simulink model "HighClearance_model"  (R2019b)
settings: configuration reference "configRef" (kept outside this file)
undefined symbols (not defined in the file): baseClearance, calSTEP1_e, calSTEP2_e, calSTEP3_e, calSTEP4_e, calTolMultiplier, errorMinSpd, heightCalibrating_e, heightDiffTolerance, heightDown_e, heightError_e, heightMovingDown_e, heightMovingUp_e, heightUnknown_e, heightUp_e, IOD_OK, IOD_Open, IOD_ScGnd, maxMedianWheelAngle, maxTransitionMachineSpd, minTransitionMachineSpd, positionSensor_tblData, positionSensorFL_BrkPnts, positionSensorFR_BrkPnts, positionSensorRL_BrkPnts, positionSensorRR_BrkPnts, step_time, trackWidthMax, trackWidthMin, trackWidthTolerance, twoWheelSteer
libraries: HighClearance_library x129, simulink x25
(part 2 of 3)

== system HighClearance_model/Inputs/clyCoilDiagsLatchLogic ==
  cylCoilDiags : Inport  OutDataTypeStr=Bus: CoilStateBus
  coilStateBreakOut : HighClearance_library/coilStateBreakOut  SystemSampleTime=-1  Latency=0  AutoFrameSizeCalculation=off
  coilStateBus : HighClearance_library/coilStateBus  SystemSampleTime=-1  Latency=0  AutoFrameSizeCalculation=off
  diagLatch{,1..7} (8 alike) : HighClearance_library/diagLatch  SystemSampleTime=-1  Latency=0  AutoFrameSizeCalculation=off
  cylCoilDiagsLatched : Outport  OutDataTypeStr=Bus: CoilStateBus
  wires:
  cylCoilDiags/1 -> coilStateBreakOut/1
  coilStateBreakOut/1 -> diagLatch/1
  diagLatch/1 -> coilStateBus/1
  coilStateBreakOut/2 -> diagLatch1/1
  diagLatch1/1 -> coilStateBus/2
  coilStateBreakOut/3 -> diagLatch2/1
  diagLatch2/1 -> coilStateBus/3
  coilStateBreakOut/5 -> diagLatch4/1
  diagLatch4/1 -> coilStateBus/5
  coilStateBreakOut/7 -> diagLatch6/1
  diagLatch6/1 -> coilStateBus/7
  coilStateBreakOut/4 -> diagLatch3/1
  coilStateBreakOut/6 -> diagLatch5/1
  coilStateBreakOut/8 -> diagLatch7/1
  diagLatch3/1 -> coilStateBus/4
  diagLatch5/1 -> coilStateBus/6
  diagLatch7/1 -> coilStateBus/8
  coilStateBus/1 -> cylCoilDiagsLatched/1

== system HighClearance_model/Inputs/legPositions ==
  positionSensors_mA : Inport  OutDataTypeStr=Bus: CylinderBus
  posSensorCalOkay : Inport  Port=2
  heightPosSensors_diag : Inport  Port=3  OutDataTypeStr=Bus: StateBus
  engRunning : Inport  Port=4  OutDataTypeStr=boolean
  Switch : Switch  Criteria=u2 > Threshold
  calibratedPositions : Subsystem
  checkPlausiLogic : Subsystem
  posSensorCalOkay1 : InportShadow  Port=2
  positionFilterLogic : HighClearance_library/positionFilterLogic  SystemSampleTime=-1  Latency=0  AutoFrameSizeCalculation=off
  positionPlausibilityCheck : Subsystem
  postionToClearance : HighClearance_library/postionToClearance  SystemSampleTime=-1  Latency=0  AutoFrameSizeCalculation=off
  uncalibratedPositions : HighClearance_library/uncalibratedPositions  SystemSampleTime=-1  Latency=0  AutoFrameSizeCalculation=off
  legClearance_mm : Outport  OutDataTypeStr=Bus: CylinderBus
  clyPositionsRaw_mm : Outport  Port=2  OutDataTypeStr=Bus: CylinderBus
  clyPositionsFlt_mm : Outport  Port=3  OutDataTypeStr=Bus: CylinderBus
  heightPosDiagsLatched : Outport  Port=4  OutDataTypeStr=Bus: StateBus
  wires:
  calibratedPositions/1(cylPos_mm) -> Switch/1
  posSensorCalOkay/1 -> Switch/2
  uncalibratedPositions/1 -> Switch/3
  Switch/1 -> positionPlausibilityCheck/2(posIn)
  positionSensors_mA/1 -> uncalibratedPositions/1, calibratedPositions/1(cylPos_mA)
  heightPosSensors_diag/1 -> postionToClearance/3
  postionToClearance/1 -> legClearance_mm/1
  positionFilterLogic/2 -> postionToClearance/1
  positionFilterLogic/1 -> clyPositionsFlt_mm/1
  postionToClearance/2 -> heightPosDiagsLatched/1
  positionPlausibilityCheck/1(posOut) -> positionFilterLogic/1, clyPositionsRaw_mm/1
  positionPlausibilityCheck/2(plausiErr) -> postionToClearance/2
  posSensorCalOkay1/1 -> checkPlausiLogic/1(posSensorCalOkay)
  engRunning/1 -> checkPlausiLogic/2(engRunning)
  checkPlausiLogic/1(enablePlausiCheck) -> positionPlausibilityCheck/1(enablePlausiCheck)

== system HighClearance_model/Inputs/trackCylCoilDiagsLatchLogic ==
  trackCylCoilDiags : Inport  OutDataTypeStr=Bus: CoilStateBus
  coilStateBreakOut : HighClearance_library/coilStateBreakOut  SystemSampleTime=-1  Latency=0  AutoFrameSizeCalculation=off
  coilStateBus : HighClearance_library/coilStateBus  SystemSampleTime=-1  Latency=0  AutoFrameSizeCalculation=off
  diagLatch{,1..7} (8 alike) : HighClearance_library/diagLatch  SystemSampleTime=-1  Latency=0  AutoFrameSizeCalculation=off
  trackCylCoilDiagsLatched : Outport  OutDataTypeStr=Bus: CoilStateBus
  wires:
  coilStateBreakOut/1 -> diagLatch/1
  diagLatch/1 -> coilStateBus/1
  coilStateBreakOut/2 -> diagLatch1/1
  diagLatch1/1 -> coilStateBus/2
  coilStateBreakOut/3 -> diagLatch2/1
  diagLatch2/1 -> coilStateBus/3
  coilStateBreakOut/5 -> diagLatch4/1
  diagLatch4/1 -> coilStateBus/5
  coilStateBreakOut/7 -> diagLatch6/1
  diagLatch6/1 -> coilStateBus/7
  coilStateBreakOut/4 -> diagLatch3/1
  coilStateBreakOut/6 -> diagLatch5/1
  coilStateBreakOut/8 -> diagLatch7/1
  diagLatch3/1 -> coilStateBus/4
  diagLatch5/1 -> coilStateBus/6
  diagLatch7/1 -> coilStateBus/8
  trackCylCoilDiags/1 -> coilStateBreakOut/1
  coilStateBus/1 -> trackCylCoilDiagsLatched/1

== system HighClearance_model/Calibration/controlLogic/calStateConverstion ==
  calState : Inport
  calState2TargetState : Stateflow chart  TreatAsAtomicUnit=on
  targetState : Outport
  wires:
  calState/1 -> calState2TargetState/1(calState)
  calState2TargetState/1(targetState) -> targetState/1

== system HighClearance_model/Calibration/controlLogic/enableCoils ==
  coilDutyCycle : Inport
  enables : Inport  Port=2  OutDataTypeStr=Bus: StateBus
  Bus Selector : BusSelector  OutputSignals=FrontLeft,FrontRight,RearLeft,RearRight
  coilBreakOut : HighClearance_library/coilBreakOut  SystemSampleTime=-1  Latency=0  AutoFrameSizeCalculation=off
  coilBus : HighClearance_library/coilBus  SystemSampleTime=-1  Latency=0  AutoFrameSizeCalculation=off
  passThroughLogic{,1..7} (8 alike) : HighClearance_library/passThroughLogic  SystemSampleTime=-1  Latency=0  AutoFrameSizeCalculation=off
  coilDutyCycle_pct : Outport  OutDataTypeStr=Bus: CoilBus
  wires:
  coilDutyCycle/1 -> coilBreakOut/1
  enables/1 -> Bus Selector/1
  coilBus/1 -> coilDutyCycle_pct/1
  coilBreakOut/1 -> passThroughLogic/1
  Bus Selector/1 -> passThroughLogic1/2, passThroughLogic/2  "<FrontLeft>"
  coilBreakOut/2 -> passThroughLogic1/1
  passThroughLogic1/1 -> coilBus/2
  passThroughLogic/1 -> coilBus/1
  passThroughLogic5/1 -> coilBus/6
  passThroughLogic6/1 -> coilBus/7
  passThroughLogic4/1 -> coilBus/5
  passThroughLogic7/1 -> coilBus/8
  passThroughLogic3/1 -> coilBus/4
  passThroughLogic2/1 -> coilBus/3
  coilBreakOut/3 -> passThroughLogic2/1
  Bus Selector/2 -> passThroughLogic3/2, passThroughLogic2/2  "<FrontRight>"
  Bus Selector/3 -> passThroughLogic5/2, passThroughLogic4/2  "<RearLeft>"
  Bus Selector/4 -> passThroughLogic6/2, passThroughLogic7/2  "<RearRight>"
  coilBreakOut/4 -> passThroughLogic3/1
  coilBreakOut/5 -> passThroughLogic4/1
  coilBreakOut/6 -> passThroughLogic5/1
  coilBreakOut/7 -> passThroughLogic6/1
  coilBreakOut/8 -> passThroughLogic7/1

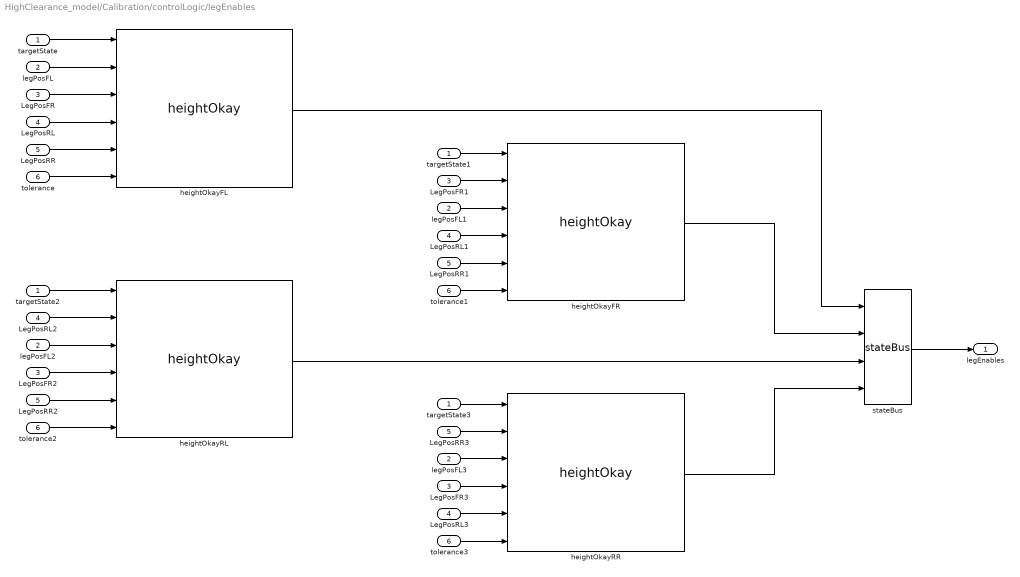
== system HighClearance_model/Calibration/controlLogic/legEnables ==
  targetState : Inport
  legPosFL : Inport  Port=2
  LegPosFR : Inport  Port=3
  LegPosRL : Inport  Port=4
  LegPosRR : Inport  Port=5
  tolerance : Inport  Port=6
  LegPosFR1 : InportShadow  Port=3
  LegPosFR2 : InportShadow  Port=3
  LegPosFR3 : InportShadow  Port=3
  LegPosRL1 : InportShadow  Port=4
  LegPosRL2 : InportShadow  Port=4
  LegPosRL3 : InportShadow  Port=4
  LegPosRR1 : InportShadow  Port=5
  LegPosRR2 : InportShadow  Port=5
  LegPosRR3 : InportShadow  Port=5
  heightOkayFL : HighClearance_library/heightOkay  SystemSampleTime=-1  Latency=0  AutoFrameSizeCalculation=off
  heightOkayFR : HighClearance_library/heightOkay  SystemSampleTime=-1  Latency=0  AutoFrameSizeCalculation=off
  heightOkayRL : HighClearance_library/heightOkay  SystemSampleTime=-1  Latency=0  AutoFrameSizeCalculation=off
  heightOkayRR : HighClearance_library/heightOkay  SystemSampleTime=-1  Latency=0  AutoFrameSizeCalculation=off
  legPosFL1 : InportShadow  Port=2
  legPosFL2 : InportShadow  Port=2
  legPosFL3 : InportShadow  Port=2
  stateBus : HighClearance_library/stateBus  SystemSampleTime=-1  Latency=0  AutoFrameSizeCalculation=off
  targetState1 : InportShadow
  targetState2 : InportShadow
  targetState3 : InportShadow
  tolerance1 : InportShadow  Port=6
  tolerance2 : InportShadow  Port=6
  tolerance3 : InportShadow  Port=6
  legEnables : Outport
  wires:
  stateBus/1 -> legEnables/1
  targetState/1 -> heightOkayFL/1
  legPosFL/1 -> heightOkayFL/2
  LegPosFR/1 -> heightOkayFL/3
  LegPosRL/1 -> heightOkayFL/4
  LegPosRR/1 -> heightOkayFL/5
  tolerance/1 -> heightOkayFL/6
  targetState1/1 -> heightOkayFR/1
  LegPosFR1/1 -> heightOkayFR/2
  legPosFL1/1 -> heightOkayFR/3
  tolerance1/1 -> heightOkayFR/6
  LegPosFR2/1 -> heightOkayRL/4
  legPosFL2/1 -> heightOkayRL/3
  targetState2/1 -> heightOkayRL/1
  tolerance2/1 -> heightOkayRL/6
  targetState3/1 -> heightOkayRR/1
  LegPosFR3/1 -> heightOkayRR/4
  LegPosRL3/1 -> heightOkayRR/5
  legPosFL3/1 -> heightOkayRR/3
  tolerance3/1 -> heightOkayRR/6
  heightOkayFL/1 -> stateBus/1
  heightOkayFR/1 -> stateBus/2
  heightOkayRL/1 -> stateBus/3
  heightOkayRR/1 -> stateBus/4
  LegPosRL1/1 -> heightOkayFR/4
  LegPosRL2/1 -> heightOkayRL/2
  LegPosRR3/1 -> heightOkayRR/2
  LegPosRR2/1 -> heightOkayRL/5
  LegPosRR1/1 -> heightOkayFR/5

== system HighClearance_model/Calibration/controlLogic/terminate1 ==
  bus : Inport
  Terminator{,1..3} (4 alike) : Terminator
  stateBreakOut : HighClearance_library/stateBreakOut  SystemSampleTime=-1  Latency=0  AutoFrameSizeCalculation=off
  wires:
  stateBreakOut/4 -> Terminator3/1
  bus/1 -> stateBreakOut/1
  stateBreakOut/3 -> Terminator2/1
  stateBreakOut/1 -> Terminator/1
  stateBreakOut/2 -> Terminator1/1

== system HighClearance_model/Calibration/controlLogic/toleranceDuringCal ==
  Constant : Constant  Value=heightDiffTolerance
  Gain : Gain  Gain=calTolMultiplier  OutDataTypeStr=Inherit: Same as input
  tolerance : Outport
  wires:
  Constant/1 -> Gain/1
  Gain/1 -> tolerance/1

== system HighClearance_model/Control/legEnablesLogic/legEnableFL ==
  targetState : Inport
  targetTrackWidth : Inport  Port=2
  actaulTrackWidth : Inport  Port=3
  legPosSubject : Inport  Port=4
  LegPosRef1 : Inport  Port=5
  LegPosRef2 : Inport  Port=6
  LegPosRef3 : Inport  Port=7
  trackCoilErrFL : Inport  Port=8
  tolerance : Inport  Port=9
  enableLogic : HighClearance_library/enableLogic  SystemSampleTime=-1  Latency=0  AutoFrameSizeCalculation=off
  heightOkay : HighClearance_library/heightOkay  SystemSampleTime=-1  Latency=0  AutoFrameSizeCalculation=off
  targetState1 : InportShadow
  targetState2 : InportShadow
  trackWidthOkay : HighClearance_library/trackWidthOkay  SystemSampleTime=-1  Latency=0  AutoFrameSizeCalculation=off
  enable : Outport
  warningTrack : Outport  Port=2
  warningHeight : Outport  Port=3
  wires:
  trackWidthOkay/1 -> enableLogic/2
  heightOkay/1 -> enableLogic/3
  enableLogic/1 -> enable/1
  enableLogic/3 -> warningHeight/1
  enableLogic/2 -> warningTrack/1
  targetState/1 -> enableLogic/1
  targetTrackWidth/1 -> trackWidthOkay/2
  actaulTrackWidth/1 -> trackWidthOkay/3
  targetState2/1 -> heightOkay/1
  targetState1/1 -> trackWidthOkay/1
  legPosSubject/1 -> heightOkay/2
  LegPosRef1/1 -> heightOkay/3
  LegPosRef2/1 -> heightOkay/4
  LegPosRef3/1 -> heightOkay/5
  tolerance/1 -> heightOkay/6
  trackCoilErrFL/1 -> trackWidthOkay/4

== system HighClearance_model/Control/legEnablesLogic/legEnableFR ==
  targetState : Inport
  targetTrackWidth : Inport  Port=2
  actaulTrackWidth : Inport  Port=3
  legPosSubject : Inport  Port=4
  LegPosRef1 : Inport  Port=5
  LegPosRef2 : Inport  Port=6
  LegPosRef3 : Inport  Port=7
  trackCoilErrFR : Inport  Port=8
  tolerance : Inport  Port=9
  enableLogic : HighClearance_library/enableLogic  SystemSampleTime=-1  Latency=0  AutoFrameSizeCalculation=off
  heightOkay : HighClearance_library/heightOkay  SystemSampleTime=-1  Latency=0  AutoFrameSizeCalculation=off
  targetState1 : InportShadow
  targetState2 : InportShadow
  trackWidthOkay : HighClearance_library/trackWidthOkay  SystemSampleTime=-1  Latency=0  AutoFrameSizeCalculation=off
  enable : Outport
  warningTrack : Outport  Port=2
  warningHeight : Outport  Port=3
  wires:
  tolerance/1 -> heightOkay/6
  LegPosRef3/1 -> heightOkay/5
  LegPosRef2/1 -> heightOkay/4
  LegPosRef1/1 -> heightOkay/3
  legPosSubject/1 -> heightOkay/2
  targetState1/1 -> trackWidthOkay/1
  targetState2/1 -> heightOkay/1
  actaulTrackWidth/1 -> trackWidthOkay/3
  targetTrackWidth/1 -> trackWidthOkay/2
  targetState/1 -> enableLogic/1
  enableLogic/2 -> warningTrack/1
  enableLogic/3 -> warningHeight/1
  enableLogic/1 -> enable/1
  trackWidthOkay/1 -> enableLogic/2
  heightOkay/1 -> enableLogic/3
  trackCoilErrFR/1 -> trackWidthOkay/4

== system HighClearance_model/Control/legEnablesLogic/legEnableRL ==
  targetState : Inport
  targetTrackWidth : Inport  Port=2
  actaulTrackWidth : Inport  Port=3
  legPosSubject : Inport  Port=4
  LegPosRef1 : Inport  Port=5
  LegPosRef2 : Inport  Port=6
  LegPosRef3 : Inport  Port=7
  trackCoilErrRL : Inport  Port=8
  tolerance : Inport  Port=9
  enableLogic : HighClearance_library/enableLogic  SystemSampleTime=-1  Latency=0  AutoFrameSizeCalculation=off
  heightOkay : HighClearance_library/heightOkay  SystemSampleTime=-1  Latency=0  AutoFrameSizeCalculation=off
  targetState1 : InportShadow
  targetState2 : InportShadow
  trackWidthOkay : HighClearance_library/trackWidthOkay  SystemSampleTime=-1  Latency=0  AutoFrameSizeCalculation=off
  enable : Outport
  warningTrack : Outport  Port=2
  warningHeight : Outport  Port=3
  wires:
  enableLogic/1 -> enable/1
  enableLogic/3 -> warningHeight/1
  enableLogic/2 -> warningTrack/1
  targetState/1 -> enableLogic/1
  targetTrackWidth/1 -> trackWidthOkay/2
  actaulTrackWidth/1 -> trackWidthOkay/3
  targetState2/1 -> heightOkay/1
  targetState1/1 -> trackWidthOkay/1
  legPosSubject/1 -> heightOkay/2
  LegPosRef1/1 -> heightOkay/3
  LegPosRef2/1 -> heightOkay/4
  LegPosRef3/1 -> heightOkay/5
  tolerance/1 -> heightOkay/6
  trackWidthOkay/1 -> enableLogic/2
  heightOkay/1 -> enableLogic/3
  trackCoilErrRL/1 -> trackWidthOkay/4

== system HighClearance_model/Control/legEnablesLogic/legEnableRR ==
  targetState : Inport
  targetTrackWidth : Inport  Port=2
  actaulTrackWidth : Inport  Port=3
  legPosSubject : Inport  Port=4
  LegPosRef1 : Inport  Port=5
  LegPosRef2 : Inport  Port=6
  LegPosRef3 : Inport  Port=7
  trackCoilErrRR : Inport  Port=8
  tolerance : Inport  Port=9
  enableLogic : HighClearance_library/enableLogic  SystemSampleTime=-1  Latency=0  AutoFrameSizeCalculation=off
  heightOkay : HighClearance_library/heightOkay  SystemSampleTime=-1  Latency=0  AutoFrameSizeCalculation=off
  targetState1 : InportShadow
  targetState2 : InportShadow
  trackWidthOkay : HighClearance_library/trackWidthOkay  SystemSampleTime=-1  Latency=0  AutoFrameSizeCalculation=off
  enable : Outport
  warningTrack : Outport  Port=2
  warningHeight : Outport  Port=3
  wires:
  tolerance/1 -> heightOkay/6
  LegPosRef3/1 -> heightOkay/5
  LegPosRef2/1 -> heightOkay/4
  LegPosRef1/1 -> heightOkay/3
  legPosSubject/1 -> heightOkay/2
  targetState1/1 -> trackWidthOkay/1
  targetState2/1 -> heightOkay/1
  actaulTrackWidth/1 -> trackWidthOkay/3
  targetTrackWidth/1 -> trackWidthOkay/2
  targetState/1 -> enableLogic/1
  enableLogic/2 -> warningTrack/1
  enableLogic/3 -> warningHeight/1
  enableLogic/1 -> enable/1
  trackWidthOkay/1 -> enableLogic/2
  heightOkay/1 -> enableLogic/3
  trackCoilErrRR/1 -> trackWidthOkay/4

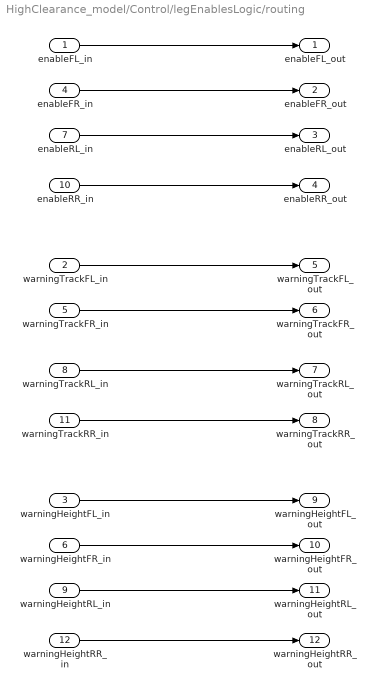
== system HighClearance_model/Control/legEnablesLogic/routing ==
  enableFL_in : Inport
  warningTrackFL_in : Inport  Port=2
  warningHeightFL_in : Inport  Port=3
  enableFR_in : Inport  Port=4
  warningTrackFR_in : Inport  Port=5
  warningHeightFR_in : Inport  Port=6
  enableRL_in : Inport  Port=7
  warningTrackRL_in : Inport  Port=8
  warningHeightRL_in : Inport  Port=9
  enableRR_in : Inport  Port=10
  warningTrackRR_in : Inport  Port=11
  warningHeightRR_in : Inport  Port=12
  enableFL_out : Outport
  enableFR_out : Outport  Port=2
  enableRL_out : Outport  Port=3
  enableRR_out : Outport  Port=4
  warningTrackFL_out : Outport  Port=5
  warningTrackFR_out : Outport  Port=6
  warningTrackRL_out : Outport  Port=7
  warningTrackRR_out : Outport  Port=8
  warningHeightFL_out : Outport  Port=9
  warningHeightFR_out : Outport  Port=10
  warningHeightRL_out : Outport  Port=11
  warningHeightRR_out : Outport  Port=12
  wires:
  enableFL_in/1 -> enableFL_out/1
  enableFR_in/1 -> enableFR_out/1
  enableRL_in/1 -> enableRL_out/1
  enableRR_in/1 -> enableRR_out/1
  warningTrackFL_in/1 -> warningTrackFL_out/1
  warningTrackFR_in/1 -> warningTrackFR_out/1
  warningTrackRL_in/1 -> warningTrackRL_out/1
  warningTrackRR_in/1 -> warningTrackRR_out/1
  warningHeightFL_in/1 -> warningHeightFL_out/1
  warningHeightFR_in/1 -> warningHeightFR_out/1
  warningHeightRL_in/1 -> warningHeightRL_out/1
  warningHeightRR_in/1 -> warningHeightRR_out/1

== system HighClearance_model/Inputs/legPositions/calibratedPositions ==
  cylPos_mA : Inport
  cylinderBreakOut : HighClearance_library/cylinderBreakOut  SystemSampleTime=-1  Latency=0  AutoFrameSizeCalculation=off
  cylinderBus : HighClearance_library/cylinderBus  SystemSampleTime=-1  Latency=0  AutoFrameSizeCalculation=off
  lookupTables : Subsystem
  cylPos_mm : Outport
  wires:
  cylPos_mA/1 -> cylinderBreakOut/1
  cylinderBus/1 -> cylPos_mm/1
  cylinderBreakOut/1 -> lookupTables/1(mA_FL)
  cylinderBreakOut/2 -> lookupTables/2(mA_FR)
  cylinderBreakOut/3 -> lookupTables/3(mA_RL)
  cylinderBreakOut/4 -> lookupTables/4(mA_RR)
  lookupTables/1(mm_FL) -> cylinderBus/1
  lookupTables/2(mm_FR) -> cylinderBus/2
  lookupTables/3(mm_RL) -> cylinderBus/3
  lookupTables/4(mm_RR) -> cylinderBus/4

== system HighClearance_model/Inputs/legPositions/checkPlausiLogic ==
  posSensorCalOkay : Inport
  engRunning : Inport  Port=2  OutDataTypeStr=boolean
  Logical Operator : Logic  AllPortsSameDT=off  OutDataTypeStr=boolean
  enablePlausiCheck : Outport
  wires:
  posSensorCalOkay/1 -> Logical Operator/2
  engRunning/1 -> Logical Operator/1
  Logical Operator/1 -> enablePlausiCheck/1

== system HighClearance_model/Inputs/legPositions/positionPlausibilityCheck ==
  enablePlausiCheck : Inport  OutDataTypeStr=boolean
  posIn : Inport  Port=2
  cylinderBreakOut : HighClearance_library/cylinderBreakOut  SystemSampleTime=-1  Latency=0  AutoFrameSizeCalculation=off
  cylinderBus : HighClearance_library/cylinderBus  SystemSampleTime=-1  Latency=0  AutoFrameSizeCalculation=off
  plausiLogic{,1..3} (4 alike) : HighClearance_library/plausiLogic  SystemSampleTime=-1  Latency=0  AutoFrameSizeCalculation=off
  stateBus : HighClearance_library/stateBus  SystemSampleTime=-1  Latency=0  AutoFrameSizeCalculation=off
  posOut : Outport
  plausiErr : Outport  Port=2
  wires:
  posIn/1 -> cylinderBreakOut/1
  cylinderBreakOut/1 -> plausiLogic/1
  plausiLogic/1 -> cylinderBus/1
  cylinderBreakOut/2 -> plausiLogic1/1
  plausiLogic1/1 -> cylinderBus/2
  cylinderBreakOut/3 -> plausiLogic2/1
  plausiLogic2/1 -> cylinderBus/3
  cylinderBreakOut/4 -> plausiLogic3/1
  plausiLogic3/1 -> cylinderBus/4
  cylinderBus/1 -> posOut/1
  stateBus/1 -> plausiErr/1
  plausiLogic/2 -> stateBus/1
  plausiLogic3/2 -> stateBus/4
  plausiLogic2/2 -> stateBus/3
  plausiLogic1/2 -> stateBus/2
  enablePlausiCheck/1 -> plausiLogic3/2, plausiLogic2/2, plausiLogic1/2, plausiLogic/2

== system HighClearance_model/Inputs/legPositions/calibratedPositions/lookupTables ==
  mA_FL : Inport
  mA_FR : Inport  Port=2
  mA_RL : Inport  Port=3
  mA_RR : Inport  Port=4
  1-D Lookup Table : Lookup_n-D  NumberOfTableDimensions=1  BreakpointsForDimension1=positionSensorFL_BrkPnts  Table=positionSensor_tblData  ExtrapMethod=Clip  UseLastTableValue=on  InternalRulePriority=Speed  RndMeth=Simplest  InputSameDT=on
  1-D Lookup Table1 : Lookup_n-D  NumberOfTableDimensions=1  BreakpointsForDimension1=positionSensorFR_BrkPnts  Table=positionSensor_tblData  ExtrapMethod=Clip  UseLastTableValue=on  InternalRulePriority=Speed  RndMeth=Simplest  InputSameDT=on
  1-D Lookup Table2 : Lookup_n-D  NumberOfTableDimensions=1  BreakpointsForDimension1=positionSensorRL_BrkPnts  Table=positionSensor_tblData  ExtrapMethod=Clip  UseLastTableValue=on  InternalRulePriority=Speed  RndMeth=Simplest  InputSameDT=on
  1-D Lookup Table3 : Lookup_n-D  NumberOfTableDimensions=1  BreakpointsForDimension1=positionSensorRR_BrkPnts  Table=positionSensor_tblData  ExtrapMethod=Clip  UseLastTableValue=on  InternalRulePriority=Speed  RndMeth=Simplest  InputSameDT=on
  mm_FL : Outport
  mm_FR : Outport  Port=2
  mm_RL : Outport  Port=3
  mm_RR : Outport  Port=4
  wires:
  mA_FL/1 -> 1-D Lookup Table/1
  mA_FR/1 -> 1-D Lookup Table1/1
  mA_RL/1 -> 1-D Lookup Table2/1
  mA_RR/1 -> 1-D Lookup Table3/1
  1-D Lookup Table/1 -> mm_FL/1
  1-D Lookup Table1/1 -> mm_FR/1
  1-D Lookup Table2/1 -> mm_RL/1
  1-D Lookup Table3/1 -> mm_RR/1

== stateflow chart HighClearance_model/Control/controlEnableLogic ==
  state disabled
    en: enable = false;
  state enabled
    en: enable = true;
  (default) -> disabled
  (junction 40) -> disabled
  (junction 29) -> (junction 40) [order 2]
  disabled -> (junction 29) [order 1] : [targetState == heightDown_e]
  (junction 29) -> enabled [order 1] : [fieldModeActive]
  (junction 31) -> (junction 29)
  disabled -> (junction 31) [order 2] : [targetState == heightUp_e]
  (junction 34) -> (junction 31)
  disabled -> (junction 34) [order 3] : [targetState == heightMovingUp_e]
  (junction 37) -> (junction 34)
  disabled -> (junction 37) [order 4] : [targetState == heightMovingDown_e]
  (junction 20) -> disabled : [targetState != heightMovingDown_e]
  (junction 22) -> (junction 20) : [targetState != heightMovingUp_e]
  (junction 15) -> (junction 22) : [targetState != heightDown_e]
  enabled -> (junction 15) [order 1] : [targetState != heightUp_e]
  enabled -> disabled [order 2] : [!fieldModeActive]
  data: fieldModeActive input; enable output boolean; targetState input; heightDown_e parameter; heightUp_e parameter; heightMovingDown_e parameter; heightMovingUp_e parameter

== stateflow chart HighClearance_model/Calibration/stateLogic/calibrationLogic ==
  state inactive
    en:
    calActive = 0;
    calOverride = 0;
    heightStop();
    clearCalValues();
    en,du:
    calState = checkCalValues();
    calOkay = checkCalOkay();
    state out = checkCalOkay [function]
      (default) -> (junction 589)
      (junction 589) -> (junction 590) [order 1] : [checkCalValues() == calOKAY_e]
      (junction 589) -> (junction 591) [order 2] : {out = false}
      (junction 590) -> (junction 592)
      (junction 592) -> (junction 591) : {out = true}
  state calCommanded
    state startConditionsFailed
      en: calState = calERROR0_e;
    state active
      en: calActive = 1; calOverride = 1; calOkay = 0;
      state updateCalDownValues [function]
        (default) -> (junction 296)
        (junction 296) -> (junction 301) : {calValues.retract.FrontLeft = mAmpFL}
        (junction 301) -> (junction 302) : {calValues.retract.FrontRight = mAmpFR}
        (junction 302) -> (junction 303) : {calValues.retract.RearLeft = mAmpRL}
        (junction 303) -> (junction 304) : {calValues.retract.RearRight = mAmpRR}
      state updateCalUpValues [function]
        (default) -> (junction 326)
        (junction 326) -> (junction 327) : {calValues.extend.FrontLeft = mAmpFL}
        (junction 327) -> (junction 328) : {calValues.extend.FrontRight = mAmpFR}
        (junction 328) -> (junction 329) : {calValues.extend.RearLeft = mAmpRL}
        (junction 329) -> (junction 330) : {calValues.extend.RearRight = mAmpRR}
      state out = doneMovingUp [function] [commented out]
        (default) -> (junction 480) [commented out]
        (junction 480) -> (junction 481) [commented out] : [legState.FrontLeft == heightUp_e || ...
            | legState.FrontLeft == heightUnknown_e]
        (junction 480) -> (junction 484) [commented out] : {out = false}
        (junction 481) -> (junction 482) [commented out] : [legState.FrontRight == heightUp_e || ...
            | legState.FrontRight == heightUnknown_e]
        (junction 482) -> (junction 483) [commented out] : [legState.RearLeft == heightUp_e || ...
            | legState.RearLeft == heightUnknown_e]
        (junction 483) -> (junction 485) [commented out] : [legState.RearRight == heightUp_e || ...
            | legState.RearRight == heightUnknown_e]
        (junction 485) -> (junction 484) [commented out] : {out = true}
      state out = pauseCal [function]
        (default) -> (junction 780)
        (junction 780) -> (junction 779) [order 1] : [(calState & calSTEP1_e) == calSTEP1_e ||...
            |  (calState & calSTEP2_e) == calSTEP2_e]
        (junction 779) -> (junction 759) : [!okayToLower]
        (junction 780) -> (junction 784) [order 2]
        (junction 759) -> (junction 778)
        (junction 784) -> (junction 782) [order 1] : [(calState & calSTEP3_e) == calSTEP3_e ||...
            |  (calState & calSTEP4_e) == calSTEP4_e]
        (junction 782) -> (junction 778) : [!okayToRaise]
        (junction 784) -> (junction 760) [order 2]
        (junction 778) -> (junction 765) : {out = true}
        (junction 760) -> (junction 765) : {out = false}
      state out = doneMovingDown [function] [commented out]
        (default) -> (junction 465) [commented out]
        (junction 465) -> (junction 466) [commented out] : [legState.FrontLeft == heightDown_e || ...
            | legState.FrontLeft == heightUnknown_e]
        (junction 465) -> (junction 469) [commented out] : {out = false}
        (junction 466) -> (junction 467) [commented out] : [legState.FrontRight == heightDown_e || ...
            | legState.FrontRight == heightUnknown_e]
        (junction 467) -> (junction 468) [commented out] : [legState.RearLeft == heightDown_e || ...
            | legState.RearLeft == heightUnknown_e]
        (junction 468) -> (junction 470) [commented out] : [legState.RearRight == heightDown_e || ...
            | legState.RearRight == heightUnknown_e]
        (junction 470) -> (junction 469) [commented out] : {out = true}
      state step3
        en: calState = calSTEP3_e;
        state active
          en: heightUp();
          state moving
          state stopped
          (default) -> calCommanded.active.step3.active.moving
          calCommanded.active.step3.active.moving -> calCommanded.active.step3.active.stopped : [checkUpValues(mAmpFL,mAmpFR,mAmpRL,mAmpRR) == calOKAY_e]
          calCommanded.active.step3.active.stopped -> calCommanded.active.step3.active.moving [order 1] : [checkUpValues(mAmpFL,mAmpFR,mAmpRL,mAmpRR) != calOKAY_e]
        state paused
          en:
          heightStop();
          calState = calState + calPAUSED_e;
          ex:
          calState = calState - calPAUSED_e;
        (default) -> calCommanded.active.step3.active
        calCommanded.active.step3.active -> calCommanded.active.step3.paused : [pauseCal()]
        calCommanded.active.step3.paused -> calCommanded.active.step3.active : [!pauseCal()]
      state step4
        en: calState = calSTEP4_e;
        state active
          en: heightUp();
        state paused
          en:
          heightStop();
          calState = calState + calPAUSED_e;
          ex:
          calState = calState - calPAUSED_e;
        (default) -> calCommanded.active.step4.active
        calCommanded.active.step4.active -> calCommanded.active.step4.paused : [pauseCal()]
        calCommanded.active.step4.paused -> calCommanded.active.step4.active : [!pauseCal()]
      state step2
        en: calState = calSTEP2_e;
        state active
          en: heightDown();
        state paused
          en:
          heightStop();
          calState = calState + calPAUSED_e;
          ex:
          calState = calState - calPAUSED_e;
        (default) -> calCommanded.active.step2.active
        calCommanded.active.step2.active -> calCommanded.active.step2.paused : [pauseCal()]
        calCommanded.active.step2.paused -> calCommanded.active.step2.active : [!pauseCal()]
      state checkDownCalValues
        en: updateCalDownValues();
        heightStop();
      state step1
        en: calState = calSTEP1_e;
        state active
          en: heightDown();
          state moving
          state stopped
          (default) -> calCommanded.active.step1.active.moving
          calCommanded.active.step1.active.moving -> calCommanded.active.step1.active.stopped : [checkDownValues(mAmpFL,mAmpFR,mAmpRL,mAmpRR) == calOKAY_e]
          calCommanded.active.step1.active.stopped -> calCommanded.active.step1.active.moving [order 1] : [checkDownValues(mAmpFL,mAmpFR,mAmpRL,mAmpRR) != calOKAY_e]
        state paused
          en:
          heightStop();
          calState = calState + calPAUSED_e;
          ex:
          calState = calState - calPAUSED_e;
        (default) -> calCommanded.active.step1.active
        calCommanded.active.step1.active -> calCommanded.active.step1.paused : [pauseCal()]
        calCommanded.active.step1.paused -> calCommanded.active.step1.active : [!pauseCal()]
      state error
        en:
        heightStop();
        state errorStep1
          en:
          calState = calERROR1_e
        state badDownCal
          en:
          calState = calERROR2_e
        state errorStep3
          en:
          calState = calERROR3_e
        state badUpCal
          en:
          calState = calERROR4_e
      state checkUpCalValues
        en: updateCalUpValues();
        heightStop();
      calCommanded.active.step3.active.stopped -> step4 [order 2] : after(calSettlingTime,msec)
      calCommanded.active.step1.active.stopped -> step2 [order 2] : after(calSettlingTime,msec)
      (default) -> step1
      step2 -> checkDownCalValues [order 1] : [calCmd == calCONFIRM2_e &&...
          | calState == calSTEP2_e]
      checkDownCalValues -> step3 [order 3] : [checkCalDownValues() == calOKAY_e]
      step2 -> step1 [order 2] : [calCmd == calDECLINE_e]
      step4 -> step3 [order 2] : [calCmd == calDECLINE_e]
      checkDownCalValues -> badDownCal [order 1] : [checkCalDownValues() == calBAD_e]
      checkDownCalValues -> badDownCal [order 2] : [!sensorsOkay() ||...
          | externalErrorActive ||...
          | !engineRunning]
      step3 -> errorStep3 [order 2] : [!sensorsOkay() ||...
          | externalErrorActive ||...
          | !engineRunning]
      step3 -> errorStep3 [order 1] : [after(calStepTimeOut,sec)]
      step4 -> checkUpCalValues [order 1] : [calCmd == calCONFIRM4_e &&...
          | calState == calSTEP4_e]
      step1 -> errorStep1 [order 2] : [!sensorsOkay() ||...
          | externalErrorActive ||...
          | !engineRunning]
      step1 -> errorStep1 [order 1] : [after(calStepTimeOut,sec)]
      checkUpCalValues -> badUpCal [order 1] : [checkCalUpValues() == calBAD_e]
      checkUpCalValues -> badUpCal [order 2] : [!sensorsOkay() ||...
          | externalErrorActive ||...
          | !engineRunning]
  state out = sensorsOkay [function]
    (default) -> (junction 829)
    (junction 829) -> (junction 830) [order 1] : [diagFL == IOD_OK]
    (junction 829) -> (junction 833) [order 2] : {out = false}
    (junction 830) -> (junction 831) : [diagFR == IOD_OK]
    (junction 831) -> (junction 832) : [diagRL == IOD_OK]
    (junction 832) -> (junction 834) : [diagRR == IOD_OK]
    (junction 834) -> (junction 833) : {out = true}
  state clearCalValues [function]
    (default) -> (junction 274) : {out = 0}
    (junction 274) -> (junction 276) : {calValues.extend.FrontLeft = out}
    (junction 276) -> (junction 277) : {calValues.extend.FrontRight  = out}
    (junction 277) -> (junction 278) : {calValues.extend.RearLeft  = out}
    (junction 278) -> (junction 279) : {calValues.extend.RearRight  = out}
    (junction 279) -> (junction 280) : {calValues.retract.FrontLeft = out}
    (junction 280) -> (junction 281) : {calValues.retract.FrontRight = out}
    (junction 281) -> (junction 282) : {calValues.retract.RearLeft = out}
    (junction 282) -> (junction 283) : {calValues.retract.RearRight = out}
  state heightStop [function]
    (default) -> (junction 154) : {outEx = 0}
    (junction 154) -> (junction 210) : {outRt = 0}
    (junction 210) -> (junction 160) : {exFL = outEx}
    (junction 160) -> (junction 168) : {exFR = outEx}
    (junction 168) -> (junction 170) : {exRL = outEx}
    (junction 170) -> (junction 173) : {exRR = outEx}
    (junction 173) -> (junction 182) : {rtFL = outRt}
    (junction 182) -> (junction 185) : {rtFR = outRt}
    (junction 185) -> (junction 186) : {rtRL = outRt}
    (junction 186) -> (junction 188) : {rtRR = outRt}
  state heightUp [function]
    (default) -> (junction 215) : {outEx = bangBang_maxOut}
    (junction 215) -> (junction 216) : {outRt = 0}
    (junction 216) -> (junction 217) : {exFL = outEx}
    (junction 217) -> (junction 218) : {exFR = outEx}
    (junction 218) -> (junction 219) : {exRL = outEx}
    (junction 219) -> (junction 220) : {exRR = outEx}
    (junction 220) -> (junction 221) : {rtFL = outRt}
    (junction 221) -> (junction 222) : {rtFR = outRt}
    (junction 222) -> (junction 223) : {rtRL = outRt}
    (junction 223) -> (junction 224) : {rtRR = outRt}
  state heightDown [function]
    (default) -> (junction 238) : {outEx = 0}
    (junction 238) -> (junction 239) : {outRt = bangBang_maxOut}
    (junction 239) -> (junction 240) : {exFL = outEx}
    (junction 240) -> (junction 241) : {exFR = outEx}
    (junction 241) -> (junction 242) : {exRL = outEx}
    (junction 242) -> (junction 243) : {exRR = outEx}
    (junction 243) -> (junction 244) : {rtFL = outRt}
    (junction 244) -> (junction 245) : {rtFR = outRt}
    (junction 245) -> (junction 246) : {rtRL = outRt}
    (junction 246) -> (junction 247) : {rtRR = outRt}
  state UpdateValues
    en: calState = calSTEP5_e;
  checkUpCalValues -> UpdateValues [order 3] : [checkCalUpValues() == calOKAY_e]
  (default) -> inactive
  (junction 107) -> startConditionsFailed
  (junction 96) -> (junction 107) [order 2]
  inactive -> (junction 96) : [hasChangedTo( calCmd, calSTART_e)]
  (junction 96) -> (junction 730) [order 1] : [okayToLower]
  (junction 730) -> (junction 842) : [okayToRaise]
  (junction 842) -> (junction 581) : [sensorsOkay()]
  (junction 581) -> (junction 853) : [!externalErrorActive]
  (junction 853) -> calCommanded.active : [engineRunning]
  UpdateValues -> inactive : after(20,msec)
  calCommanded -> inactive : [calCmd == calABORT_e]
  data: state function_output uint16; out function_output boolean; out function_output boolean; out function_output boolean; out function_output boolean; out function_output boolean; state function_output uint16; state function_output uint16; out local single; outEx temporary single; outRt temporary single; outEx temporary single; outRt temporary single; outEx temporary single; outRt temporary single; state function_output uint16; FL function_input single; FR function_input single; RL function_input single; RR function_input single; state function_output uint16; FL function_input single; FR function_input single; RL function_input single; RR function_input single; engineRunning input; calActive output boolean; calOkay output boolean; calOverride output boolean; exFL output single; rtFL output single; exFR output single; rtFR output single; exRL output single; rtRL output single; exRR output single; rtRR output single; calState output uint16; calCmd input uint16; mAmpFL input single; mAmpFR input single; mAmpRL input single; mAmpRR input single; diagFL input uint8; diagFR input uint8; diagRL input uint8; diagRR input uint8; calSTART_e parameter; calSTEP1_e parameter; calSTEP2_e parameter; calCONFIRM2_e parameter; calSTEP3_e parameter; calSTEP4_e parameter; calCONFIRM4_e parameter; calABORT_e parameter; calDECLINE_e parameter; calERROR0_e parameter; calERROR1_e parameter; calERROR2_e parameter; calERROR3_e parameter; calERROR4_e parameter; calBAD_e parameter; calSensorTolerance parameter; positionSensorFL_BrkPnts parameter; defaultPositionSensor_BrkPnts parameter; calOKAY_e parameter; positionSensorFR_BrkPnts parameter; positionSensorRL_BrkPnts parameter; positionSensorRR_BrkPnts parameter; calValues output Bus: CoilBus; IOD_OK parameter; calStepTimeOut parameter; legState input Bus: StateBus; heightUp_e parameter; heightDown_e parameter; calSettlingTime parameter; heightUnknown_e parameter; externalErrorActive input; okayToRaise input; okayToLower input; calSTEP5_e parameter; bangBang_maxOut parameter; calPAUSED_e parameter
  function state = checkCalValues:
    | function state = checkCalValues
    | 
    | state = calBAD_e;
    | 
    | if 	positionSensorFL_BrkPnts(1) > ( defaultPositionSensor_BrkPnts(1) - calSensorTolerance ) && ...
    | 	positionSensorFL_BrkPnts(1) < ( defaultPositionSensor_BrkPnts(1) + calSensorTolerance ) && ...
    |     positionSensorFL_BrkPnts(2) > ( defaultPositionSensor_BrkPnts(2) - calSensorTolerance ) && ...
    |     positionSensorFL_BrkPnts(2) < ( defaultPositionSensor_BrkPnts(2) + calSensorTolerance )
    |     
    |     if 	positionSensorFR_BrkPnts(1) > ( defaultPositionSensor_BrkPnts(1) - calSensorTolerance ) && ...
    |         positionSensorFR_BrkPnts(1) < ( defaultPositionSensor_BrkPnts(1) + calSensorTolerance ) && ...
    |         positionSensorFR_BrkPnts(2) > ( defaultPositionSensor_BrkPnts(2) - calSensorTolerance ) && ...
    |         positionSensorFR_BrkPnts(2) < ( defaultPositionSensor_BrkPnts(2) + calSensorTolerance )
    |     
    |         if 	positionSensorRL_BrkPnts(1) > ( defaultPositionSensor_BrkPnts(1) - calSensorTolerance ) && ...
    |             positionSensorRL_BrkPnts(1) < ( defaultPositionSensor_BrkPnts(1) + calSensorTolerance ) && ...
    |             positionSensorRL_BrkPnts(2) > ( defaultPositionSensor_BrkPnts(2) - calSensorTolerance ) && ...
    |             positionSensorRL_BrkPnts(2) < ( defaultPositionSensor_BrkPnts(2) + calSensorTolerance )
    |         
    |             if 	positionSensorRR_BrkPnts(1) > ( defaultPositionSensor_BrkPnts(1) - calSensorTolerance ) && ...
    |                 positionSensorRR_BrkPnts(1) < ( defaultPositionSensor_BrkPnts(1) + calSensorTolerance ) && ...
    |                 positionSensorRR_BrkPnts(2) > ( defaultPositionSensor_BrkPnts(2) - calSensorTolerance ) && ...
    |                 positionSensorRR_BrkPnts(2) < ( defaultPositionSensor_BrkPnts(2) + calSensorTolerance )
    |             
    |                 state = calOKAY_e;
    | 
    |             end
    | 
    |         end
    |         
    |     end
    |     
    | end
    |  
    | end
  function state = checkCalDownValues:
    | function state = checkCalDownValues
    | 
    |     state = checkDownValues(calValues.retract.FrontLeft,...
    |         calValues.retract.FrontRight,...
    |         calValues.retract.RearLeft,...
    |         calValues.retract.RearRight);
    | 
    | end
  function state = checkCalUpValues:
    | function state = checkCalUpValues
    | 
    |     state = checkUpValues(calValues.extend.FrontLeft,...
    |         calValues.extend.FrontRight,...
    |         calValues.extend.RearLeft,...
    |         calValues.extend.RearRight);
    | 
    | end
  function state = checkDownValues(FL, FR, RL, RR):
    | function state = checkDownValues(FL, FR, RL, RR)
    | 
    | state = calBAD_e;
    | 
    | if 	FL > ( defaultPositionSensor_BrkPnts(1) - calSensorTolerance ) && ...
    |     FL < ( defaultPositionSensor_BrkPnts(1) + calSensorTolerance )
    |     
    |     if 	FR > ( defaultPositionSensor_BrkPnts(1) - calSensorTolerance ) && ...
    |         FR < ( defaultPositionSensor_BrkPnts(1) + calSensorTolerance )
    |     
    |         if 	RL > ( defaultPositionSensor_BrkPnts(1) - calSensorTolerance ) && ...
    |             RL < ( defaultPositionSensor_BrkPnts(1) + calSensorTolerance )
    |         
    |             if 	RR > ( defaultPositionSensor_BrkPnts(1) - calSensorTolerance ) && ...
    |                 RR < ( defaultPositionSensor_BrkPnts(1) + calSensorTolerance )
    |             
    |                 state = calOKAY_e;
    | 
    |             end
    | 
    |         end
    |         
    |     end
    |     
    | end
    |  
    | end
  function state = checkUpValues(FL, FR, RL ,RR):
    | function state = checkUpValues(FL, FR, RL ,RR)
    | 
    | state = calBAD_e;
    | 
    | if 	FL > ( defaultPositionSensor_BrkPnts(2) - calSensorTolerance ) && ...
    |     FL < ( defaultPositionSensor_BrkPnts(2) + calSensorTolerance )
    |     
    |     if 	FR > ( defaultPositionSensor_BrkPnts(2) - calSensorTolerance ) && ...
    |         FR < ( defaultPositionSensor_BrkPnts(2) + calSensorTolerance )
    |     
    |         if 	RL > ( defaultPositionSensor_BrkPnts(2) - calSensorTolerance ) && ...
    |             RL < ( defaultPositionSensor_BrkPnts(2) + calSensorTolerance )
    |         
    |             if 	RR > ( defaultPositionSensor_BrkPnts(2) - calSensorTolerance ) && ...
    |                 RR < ( defaultPositionSensor_BrkPnts(2) + calSensorTolerance )
    |             
    |                 state = calOKAY_e;
    | 
    |             end
    | 
    |         end
    |         
    |     end
    |     
    | end
    |  
    | end

== stateflow chart HighClearance_model/Arbitration/TargetPositionArbitration/TargetPosition ==
  state positionStates
    state up
      en:
      targetPos.FrontLeft = positionSensor_tblData[1] + baseClearance;
      targetPos.FrontRight = positionSensor_tblData[1] + baseClearance;
      targetPos.RearLeft = positionSensor_tblData[1] + baseClearance;
      targetPos.RearRight = positionSensor_tblData[1] + baseClearance;
    state down
      en:
      targetPos.FrontLeft = positionSensor_tblData[0] + baseClearance;
      targetPos.FrontRight = positionSensor_tblData[0] + baseClearance;
      targetPos.RearLeft = positionSensor_tblData[0] + baseClearance;
      targetPos.RearRight = positionSensor_tblData[0] + baseClearance;
    state stop
      en,du:
      targetPos.FrontLeft = cylPosFL;
      targetPos.FrontRight = cylPosFR;
      targetPos.RearLeft = cylPosRL;
      targetPos.RearRight = cylPosRR;
    (default) -> (junction 20)
    (junction 20) -> up [order 1] : [targetState == heightUp_e ||...
        | targetState == heightMovingUp_e]
    (junction 20) -> down [order 2] : [targetState == heightDown_e ||...
        | targetState == heightMovingDown_e]
    (junction 20) -> stop [order 3]
  positionStates -> positionStates : [hasChanged(targetState)]
  (default) -> positionStates
  data: targetState input; positionSensor_tblData parameter; heightDown_e parameter; heightUp_e parameter; heightMovingUp_e parameter; heightMovingDown_e parameter; heightCalibrating_e parameter; heightError_e parameter; heightUnknown_e parameter; cylPosFL input single; cylPosFR input single; cylPosRL input single; cylPosRR input single; targetPos output Bus: CylinderBus =0; baseClearance parameter
